simulink model "SguanFOC"  (R2025a)
settings: Solver=FixedStepAuto  StartTime=0.0  StopTime=5  FixedStep=0.00001  RelTol=1e-3
InitFcn:
  | T = 0.0001;
  | VBUS = 311;
  | 
  | Ld = 0.00525;
  | Lq = 0.012;
  | Rs = 0.958;
  | 
  | 
  | Wc = 1000;
  | Ws = 8;
  | 
  | W_b = 2000;
undefined symbols (not defined in the file): DiscIntNeverNeededParam, Down, Up
libraries: eePwmGenerator x3, powerlib_extras x2, spsDCVoltageSourceLib x1, spsPermanentMagnetSynchronousMachineLib x1, spsSawtoothGeneratorLib x1, spsUniversalBridgeLib x1, spspowerguiLib x1
settings Model: Creator=星必尘Sguan  LastModifiedBy=星必尘Sguan
settings SFSimCC: SimCustomHeaderCode="#include \"SVPWM.h\""  SimUserSources=SVPWM.c

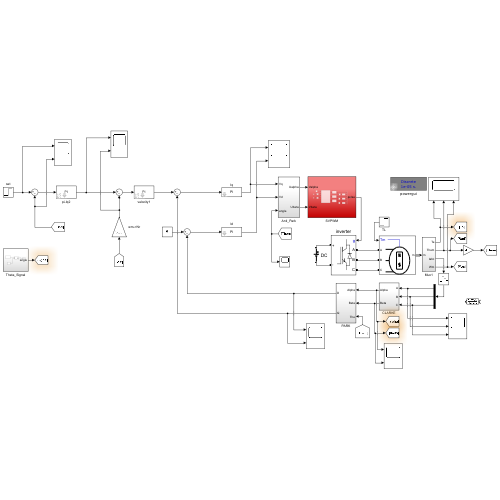
[thumbnail: Simulink's stored preview of the top-level diagram]
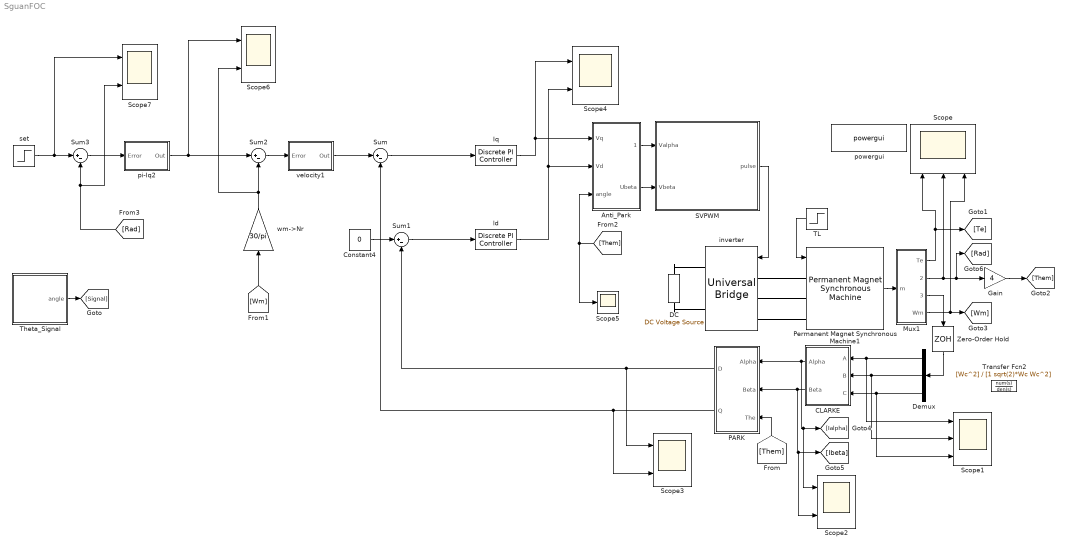
== system SguanFOC ==
  Anti_Park : Subsystem
  CLARKE : Subsystem
  Constant4 : Constant  Value=0
  DC : spsDCVoltageSourceLib/DC Voltage Source  Amplitude=VBUS  Measurements=Voltage
  Demux : Demux  Outputs=3
  Gain : Gain  Gain=4
  Iq : powerlib_extras/Discrete  Control Blocks/Discrete PI Controller  Kp=40  Ki=3193.3  Par_Limits=[340*0.9*sqrt(1/3) -340*0.9*sqrt(1/3)]  Init=0  Ts=1e-4
  Mux1 : Subsystem
  PARK : Subsystem
  Permanent Magnet Synchronous Machine1 : spsPermanentMagnetSynchronousMachineLib/Permanent Magnet Synchronous Machine  NbPhases=3  FluxDistribution=Sinusoidal  RotorType=Salient-pole  MechanicalLoad=Torque Tm  PresetModel=No  ShowDetailedParameters=on  MeasurementBus=off  Resistance=0.958  Inductance=8.5e-3  dqInductances=[5.25e-3,12e-3]  La=0.000835  MachineConstant=Flux linkage established by magnets (V.s)  Flux=0.1827  VoltageCst=132.5525  TorqueCst=1.0962  Flat=120  Mechanical=[0.003 0.008 4]  PolePairs=3  InitialConditions=[0,0, 0,0]  InitialConditions5ph=[0 0 0 0 0 0]  RefAngle=Aligned with phase A axis (original Park)  IterativeDiscreteModel=Trapezoidal non iterative  TsBlock=-1  TsPowergui=0
  SVPWM : Subsystem
  Scope : Scope  NumInputPorts=3
      settings: ActiveDisplayYMinimum=71.221659633413722  ActiveDisplayYMaximum=83.45959853190611
  Scope1 : Scope  NumInputPorts=3
      settings: ActiveDisplayYMinimum=-56.765093426646764  ActiveDisplayYMaximum=56.919768702194638
  Scope{2..4,6..7} (5 alike) : Scope  NumInputPorts=2
      Scope2 settings: ActiveDisplayYMinimum=-3.4308453898305751  ActiveDisplayYMaximum=14.952214172172493  DataLoggingVariableName=ScopeData2
      Scope3 settings: ActiveDisplayYMinimum=-12.718687980408173  ActiveDisplayYMaximum=11.569758124701689  DataLoggingVariableName=ScopeData3
      Scope4 settings: ActiveDisplayYMinimum=-120.45590110912798  ActiveDisplayYMaximum=249.87801666414541  DataLoggingVariableName=ScopeData4
      Scope6 settings: ActiveDisplayYMinimum=-6.298375426201801  ActiveDisplayYMaximum=1828.1288182778874  DataLoggingVariableName=ScopeData6
      Scope7 settings: ActiveDisplayYMinimum=3.84321816794486  ActiveDisplayYMaximum=20.129691037464234  DataLoggingVariableName=ScopeData7
  Scope5 : Scope
      settings: ActiveDisplayYMinimum=-2.417785617585527  ActiveDisplayYMaximum=0.38689833522072209  DataLoggingVariableName=ScopeData5
  Sum{,1..3} (4 alike) : Sum  Inputs=|+-
  TL : Step  Time=3  SampleTime=0
  Theta_Signal : Subsystem
  Transfer Fcn2 : TransferFcn  Numerator=[Wc^2]  Denominator=[1 sqrt(2)*Wc Wc^2]
  Zero-Order Hold : ZeroOrderHold  SampleTime=0.0001
  inverter : spsUniversalBridgeLib/Universal Bridge  Arms=3  SnubberResistance=1e5  SnubberCapacitance=inf  Device=IGBT / Diodes  Ron=1e-3  Lon=0  ForwardVoltages="[  0  0  ]"  ForwardVoltage=0  GTOparameters=[ 10e-6 , 20e-6 ]  IGBTparameters=[ 1e-6 , 2e-6 ]  Measurements=None  Measurements_2=None  converterType=Rectifier
  ld : powerlib_extras/Discrete  Control Blocks/Discrete PI Controller  Kp=17.5  Ki=3193.3  Par_Limits=[340*0.9*sqrt(1/3) -340*0.9*sqrt(1/3)]  Init=0  Ts=0.0001
  pi-Iq2 : Subsystem  AncestorBlock=|  DialogController=POWERSYS.PowerSysDialog  mask(Discrete PI Controller){Kp=270, Ki=0, Par_Limits=[2500 -2500], Init=0, Ts=2.5e-3}
      | powerlib_extras/Discrete 
      | Control Blocks/Discrete
      | PI Controller
      mask prompts: Kp "Proportional gain (Kp):"; Ki "Integral gain (Ki):"; Par_Limits "Output limits: [ Upper   Lower ]"; Init "Output initial value:"; Ts "Sample time:"
      mask help: This block implements a discrete PI controller.
      mask init:
      | UpperLimit=Par_Limits(1);
      | LowerLimit=Par_Limits(2);
      | power_initmask();
      mask Help: This block is part of a subset of blocks in the Extras library that does not have documentation associated with it, other than the block mask description.
      mask Display: disp('PI');
  powergui : spspowerguiLib/powergui  SimulationMode=Discrete  SampleTime=1e-5  frequency=60  Iterations=50  frequencyindice=0  Pbase=100e6  ErrMax=1e-4  UnitsV=kV  UnitsW=MW  buscounter=0  FunctionMessages=off  echomessages=off  EnableUseOfTLC=off  CurrentSourceSwitches=off  DisableSnubberDevices=off  DisableRonSwitches=off  DisableVfSwitches=off  DisplayEquations=off  AutomaticDiscreteSolvers=off  SolverType=Tustin/Backward Euler (TBE)  Interpol=off  ExternalGateDelay=off  methode=off  Ts=0  x0status=blocks  SPID=off  SwTol=0  HookPort=off  NonlinearTolerance=1e-4  nMaxIteration=100  ContinueOnMaxIteration=off  RestoreLinks=warning  ResistiveCurrentMeasurement=off  Frange=[0:2:500]  Ylog=off  Xlog=on  ShowGrid=off  save=off  variable=ZData  structure=0  ZoomFFT=on  StartTime=0.0  cycles=1  DisplayStyle=1  fundamental=60  FreqAxis=off  MaxFrequency=1000  frequencyindicesteady=1  RmsSteady=1  display=off
  set : Step  Time=2  After=20  SampleTime=0
  velocity1 : Subsystem  AncestorBlock=|  DialogController=POWERSYS.PowerSysDialog  mask(Discrete PI Controller){Kp=0.0294, Ki=1.472, Par_Limits=[20 -20], Init=0, Ts=5e-4}
      | powerlib_extras/Discrete 
      | Control Blocks/Discrete
      | PI Controller
      mask prompts: Kp "Proportional gain (Kp):"; Ki "Integral gain (Ki):"; Par_Limits "Output limits: [ Upper   Lower ]"; Init "Output initial value:"; Ts "Sample time:"
      mask help: This block implements a discrete PI controller.
      mask init:
      | UpperLimit=Par_Limits(1);
      | LowerLimit=Par_Limits(2);
      | power_initmask();
      mask Help: This block is part of a subset of blocks in the Extras library that does not have documentation associated with it, other than the block mask description.
      mask Display: disp('PI');
  wm->Nr : Gain  Gain=30/pi
  wires:
  Permanent Magnet Synchronous Machine1/1 -> Mux1/1(m)
  Mux1/3(Iabc) -> Zero-Order Hold/1
  Theta_Signal/1(angle) -> [Signal]
  Sum1/1 -> ld/1
  CLARKE/1(Alpha) -> PARK/1(Alpha), Scope2/1, [Ialpha]
  CLARKE/2(Beta) -> PARK/2(Beta), Scope2/2, [Ibeta]
  Mux1/1(Te) -> Scope/1, [Te]
  Mux1/4(Wm) -> [Wm], Scope/3
  [Them] -> PARK/3(The)
  PARK/1(D) -> Scope3/1, Sum1/2
  PARK/2(Q) -> Scope3/2, Sum/2
  Constant4/1 -> Sum1/1
  [Them] -> Scope5/1, Anti_Park/3(angle)
  Zero-Order Hold/1 -> Demux/1
  Sum/1 -> Iq/1
  Anti_Park/1(Ualpha) -> SVPWM/1(Valpha)
  Anti_Park/2(Ubeta) -> SVPWM/2(Vbeta)
  SVPWM/1(pulse) -> inverter/1
  Iq/1 -> Anti_Park/1(Vq), Scope4/1
  ld/1 -> Scope4/2, Anti_Park/2(Vd)
  Mux1/2(Them) -> [Rad], Gain/1, Scope/2
  Gain/1 -> [Them]
  Demux/1 -> Scope1/1, CLARKE/1(A)
  Demux/2 -> Scope1/2, CLARKE/2(B)
  Demux/3 -> Scope1/3, CLARKE/3(C)
  [Wm] -> wm->Nr/1
  wm->Nr/1 -> Scope6/2, Sum2/2
  TL/1 -> Permanent Magnet Synchronous Machine1/1
  velocity1/1(Out) -> Sum/1
  Sum2/1 -> velocity1/1(Error)
  pi-Iq2/1(Out) -> Scope6/1, Sum2/1
  Sum3/1 -> pi-Iq2/1(Error)
  set/1 -> Scope7/1, Sum3/1
  [Rad] -> Scope7/2, Sum3/2
  connections:
  DC/RConn1 -- inverter/RConn1
  DC/LConn1 -- inverter/RConn2
  inverter/LConn1 -- Permanent Magnet Synchronous Machine1/LConn1
  Permanent Magnet Synchronous Machine1/LConn2 -- inverter/LConn2
  Permanent Magnet Synchronous Machine1/LConn3 -- inverter/LConn3

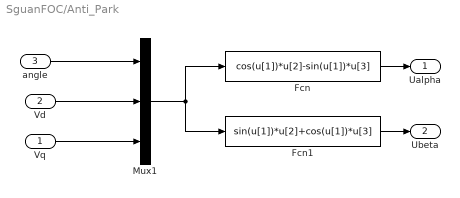
== system SguanFOC/Anti_Park ==
  Vq : Inport
  Vd : Inport  Port=2
  angle : Inport  Port=3
  Fcn : Fcn  Expr=cos(u[1])*u[2]-sin(u[1])*u[3]
  Fcn1 : Fcn  Expr=sin(u[1])*u[2]+cos(u[1])*u[3]
  Mux1 : Mux  Inputs=3
  Ualpha : Outport
  Ubeta : Outport  Port=2
  wires:
  angle/1 -> Mux1/1
  Vq/1 -> Mux1/3
  Vd/1 -> Mux1/2
  Mux1/1 -> Fcn1/1, Fcn/1
  Fcn/1 -> Ualpha/1
  Fcn1/1 -> Ubeta/1

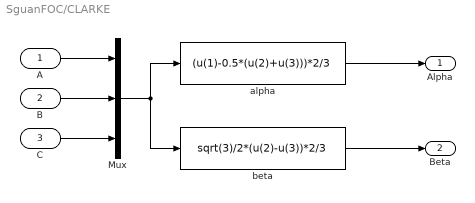
== system SguanFOC/CLARKE ==
  A : Inport
  B : Inport  Port=2
  C : Inport  Port=3
  Mux : Mux  Inputs=3
  alpha : Fcn  Expr=(u(1)-0.5*(u(2)+u(3)))*2/3
  beta : Fcn  Expr=sqrt(3)/2*(u(2)-u(3))*2/3
  Alpha : Outport
  Beta : Outport  Port=2
  wires:
  beta/1 -> Beta/1
  Mux/1 -> alpha/1, beta/1
  A/1 -> Mux/1
  C/1 -> Mux/3
  B/1 -> Mux/2
  alpha/1 -> Alpha/1

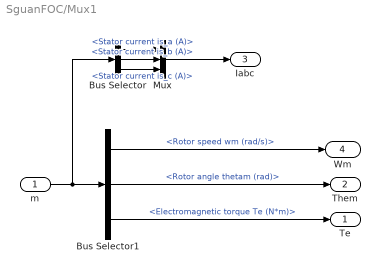
== system SguanFOC/Mux1 ==
  m : Inport
  Bus Selector : BusSelector  OutputSignals=Stator current is_a (A),Stator current is_b (A),Stator current is_c (A)
  Bus Selector1 : BusSelector  OutputSignals=Rotor speed wm (rad/s),Rotor angle thetam (rad),Electromagnetic torque Te (N*m)
  Mux : Mux  Inputs=3
  Te : Outport
  Them : Outport  Port=2
  Iabc : Outport  Port=3
  Wm : Outport  Port=4
  wires:
  Bus Selector1/2 -> Them/1  "<Rotor angle thetam (rad)>"
  Bus Selector1/3 -> Te/1  "<Electromagnetic torque Te (N*m)>"
  m/1 -> Bus Selector/1, Bus Selector1/1
  Bus Selector/2 -> Mux/2  "<Stator current is_b (A)>"
  Bus Selector/3 -> Mux/3  "<Stator current is_c (A)>"
  Bus Selector/1 -> Mux/1  "<Stator current is_a (A)>"
  Mux/1 -> Iabc/1
  Bus Selector1/1 -> Wm/1  "<Rotor speed wm (rad/s)>"

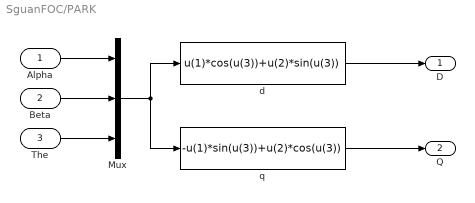
== system SguanFOC/PARK ==
  Alpha : Inport
  Beta : Inport  Port=2
  The : Inport  Port=3
  Mux : Mux  Inputs=3
  d : Fcn  Expr=u(1)*cos(u(3))+u(2)*sin(u(3))
  q : Fcn  Expr=-u(1)*sin(u(3))+u(2)*cos(u(3))
  D : Outport
  Q : Outport  Port=2
  wires:
  The/1 -> Mux/3
  q/1 -> Q/1
  Mux/1 -> d/1, q/1
  Alpha/1 -> Mux/1
  Beta/1 -> Mux/2
  d/1 -> D/1

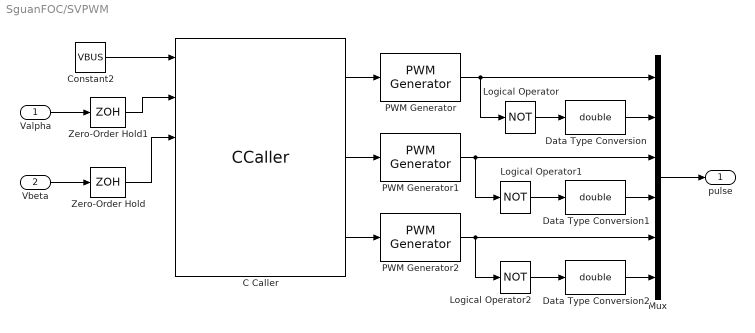
== system SguanFOC/SVPWM ==
  Valpha : Inport
  Vbeta : Inport  Port=2
  C Caller : CCaller  FunctionName=SVPWM  PortSpecificationStruct="%)30     .    8 H   8    (     @         %    \"     8    !     0         %  0 \"0    $    _    07)G3F%M90  4&]R=$YA;64 4V-O<&4     26YD97@     5'EP90      4VEZ90      27-';&]B86P   X    P    !@    @    $          4    (     0    0    !         !  ! !60E53#@   #     &    \"     0         !0    @    !    !     $         $  $ %9\"55,.    .     8    (    !          %    \"     $    %     0         0  ...(+3198 chars)"
  Constant2 : Constant  Value=VBUS
  Data Type Conversion : DataTypeConversion  OutDataTypeStr=double  SaturateOnIntegerOverflow=off  RndMeth=Floor
  Data Type Conversion1 : DataTypeConversion  OutDataTypeStr=double  SaturateOnIntegerOverflow=off  RndMeth=Floor
  Data Type Conversion2 : DataTypeConversion  OutDataTypeStr=double  SaturateOnIntegerOverflow=off  RndMeth=Floor
  Logical Operator : Logic  Operator=NOT  AllPortsSameDT=off  OutDataTypeStr=boolean
  Logical Operator1 : Logic  Operator=NOT  AllPortsSameDT=off  OutDataTypeStr=boolean
  Logical Operator2 : Logic  Operator=NOT  AllPortsSameDT=off  OutDataTypeStr=boolean
  Mux : Mux  Inputs=6
  PWM Generator : eePwmGenerator/PWM Generator  CarrCount=Up-Down  Tper=0.0001  Tdelay=0  Ts=1e-5
  PWM Generator1 : eePwmGenerator/PWM Generator  CarrCount=Up-Down  Tper=0.0001  Tdelay=0  Ts=1e-5
  PWM Generator2 : eePwmGenerator/PWM Generator  CarrCount=Up-Down  Tper=0.0001  Tdelay=0  Ts=1e-5
  Zero-Order Hold : ZeroOrderHold  SampleTime=T
  Zero-Order Hold1 : ZeroOrderHold  SampleTime=T
  pulse : Outport
  wires:
  Data Type Conversion2/1 -> Mux/6
  Logical Operator2/1 -> Data Type Conversion2/1
  PWM Generator/1 -> Mux/1, Logical Operator/1
  C Caller/1 -> PWM Generator/1
  Logical Operator1/1 -> Data Type Conversion1/1
  Constant2/1 -> C Caller/1
  Zero-Order Hold1/1 -> C Caller/2
  Data Type Conversion/1 -> Mux/2
  Data Type Conversion1/1 -> Mux/4
  Mux/1 -> pulse/1
  Zero-Order Hold/1 -> C Caller/3
  PWM Generator2/1 -> Logical Operator2/1, Mux/5
  PWM Generator1/1 -> Logical Operator1/1, Mux/3
  Logical Operator/1 -> Data Type Conversion/1
  Vbeta/1 -> Zero-Order Hold/1
  C Caller/2 -> PWM Generator1/1
  C Caller/3 -> PWM Generator2/1
  Valpha/1 -> Zero-Order Hold1/1

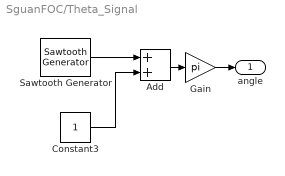
== system SguanFOC/Theta_Signal ==
  Add : Sum
  Constant3 : Constant
  Gain : Gain  Gain=pi
  Sawtooth Generator : spsSawtoothGeneratorLib/Sawtooth Generator  Freq=10  Phase=180  Ts=0
  angle : Outport
  wires:
  Add/1 -> Gain/1
  Constant3/1 -> Add/2
  Gain/1 -> angle/1
  Sawtooth Generator/1 -> Add/1

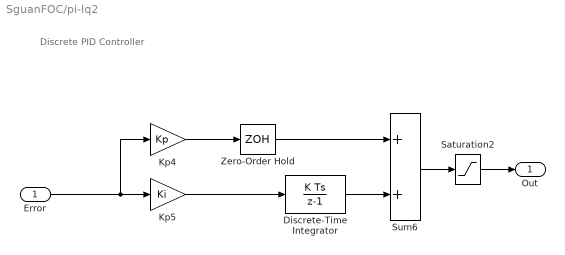
== system SguanFOC/pi-Iq2 ==
  note: Discrete PID Controller
  Error : Inport  SampleTime=Ts
  Discrete-Time Integrator : DiscreteIntegrator  InitialCondition=Init  SampleTime=Ts  LimitOutput=on  UpperSaturationLimit=UpperLimit  LowerSaturationLimit=LowerLimit  ICPrevOutput=DiscIntNeverNeededParam  ICPrevScaledInput=DiscIntNeverNeededParam
  Kp4 : Gain  Gain=Kp  SaturateOnIntegerOverflow=on  SampleTime=Ts  OutDataTypeStr=Inherit: Same as input  ParamDataTypeStr=Inherit: Same as input
  Kp5 : Gain  Gain=Ki  SaturateOnIntegerOverflow=on  SampleTime=Ts  OutDataTypeStr=Inherit: Same as input  ParamDataTypeStr=Inherit: Same as input
  Saturation2 : Saturate  UpperLimit=UpperLimit  LowerLimit=LowerLimit  SampleTime=Ts
  Sum6 : Sum  InputSameDT=on  SaturateOnIntegerOverflow=on  SampleTime=Ts  OutDataTypeStr=Inherit: Same as first input
  Zero-Order Hold : ZeroOrderHold  SampleTime=Ts
  Out : Outport  SampleTime=Ts  InitialOutput=0
  wires:
  Error/1 -> Kp4/1, Kp5/1
  Sum6/1 -> Saturation2/1
  Kp5/1 -> Discrete-Time Integrator/1
  Kp4/1 -> Zero-Order Hold/1
  Discrete-Time Integrator/1 -> Sum6/2
  Saturation2/1 -> Out/1
  Zero-Order Hold/1 -> Sum6/1

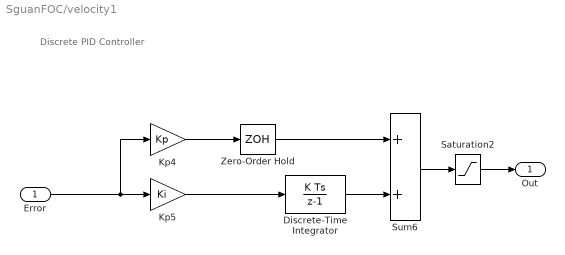
== system SguanFOC/velocity1 ==
  note: Discrete PID Controller
  Error : Inport  SampleTime=Ts
  Discrete-Time Integrator : DiscreteIntegrator  InitialCondition=Init  SampleTime=Ts  LimitOutput=on  UpperSaturationLimit=UpperLimit  LowerSaturationLimit=LowerLimit  ICPrevOutput=DiscIntNeverNeededParam  ICPrevScaledInput=DiscIntNeverNeededParam
  Kp4 : Gain  Gain=Kp  SaturateOnIntegerOverflow=on  SampleTime=Ts  OutDataTypeStr=Inherit: Same as input  ParamDataTypeStr=Inherit: Same as input
  Kp5 : Gain  Gain=Ki  SaturateOnIntegerOverflow=on  SampleTime=Ts  OutDataTypeStr=Inherit: Same as input  ParamDataTypeStr=Inherit: Same as input
  Saturation2 : Saturate  UpperLimit=UpperLimit  LowerLimit=LowerLimit  SampleTime=Ts
  Sum6 : Sum  InputSameDT=on  SaturateOnIntegerOverflow=on  SampleTime=Ts  OutDataTypeStr=Inherit: Same as first input
  Zero-Order Hold : ZeroOrderHold  SampleTime=Ts
  Out : Outport  SampleTime=Ts  InitialOutput=0
  wires:
  Error/1 -> Kp4/1, Kp5/1
  Sum6/1 -> Saturation2/1
  Kp5/1 -> Discrete-Time Integrator/1
  Kp4/1 -> Zero-Order Hold/1
  Discrete-Time Integrator/1 -> Sum6/2
  Saturation2/1 -> Out/1
  Zero-Order Hold/1 -> Sum6/1
